simulink model "Imduction_Motor_Model_main"  (R2024a)
settings: Solver=VariableStepAuto  StartTime=0.0  StopTime=15  RelTol=1e-3
libraries: POWER_FACTOR x2, spsPower3phInstantaneousLib x2, spsThreePhaseVIMeasurementLib x2, spsAsynchronousMachineSIUnitsLib x1, Auto_transformer_Starter x1, spsGroundLib x1, Over_Voltage_Protection_Relay x1, Over_Current_Protection_Relay x1, Random_Torque_signal_Generator x1, spsThreePhaseProgrammableVoltageSourceLib x1, spspowerguiLib x1
settings Model: Creator=gshma  LastModifiedBy=gshma

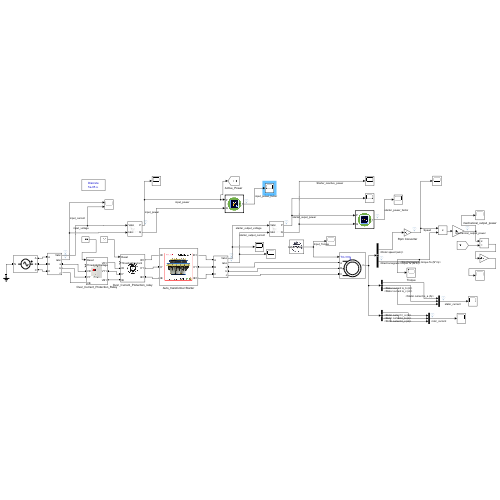
[thumbnail: Simulink's stored preview of the top-level diagram]
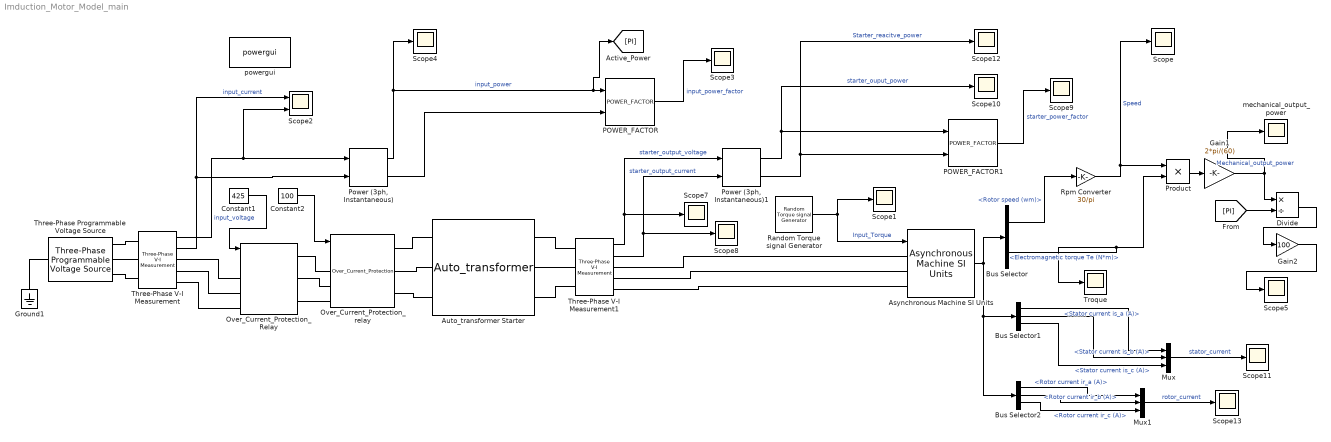
== system Imduction_Motor_Model_main ==
  Asynchronous Machine SI Units : spsAsynchronousMachineSIUnitsLib/Asynchronous Machine SI Units  RotorType=Squirrel-cage  PresetModel="15:  5.4 HP (4KW)   400 V  50Hz 1430 RPM"  MechanicalLoad=Torque Tm  ShowDetailedParameters=on  ReferenceFrame=Rotor  Units=SI  MeasurementBus=off  NominalParameters=[4000 400 50]  VoltageRatio=1  Stator=[1.405 0.005839]  Rotor=[1.395 0.005839]  Cage1=[0.4155 0.002066]  Cage2=[0.4168 0.0003495]  Lm=0.1722  Mechanical=[0.0131 0.002985 2]  PolePairs=2  InitialConditions=[0.05 0 0 0 0 0 0 0]  SimulateSaturation=off  Saturation=[14.03593122, 27.81365428, 53.79336849, 72.68890987, 97.98006896, 148.6815601, 215.7428561, 302.9841135, 428.7778367 ; 230, 322, 414, 460, 506, 552, 598, 644, 690]  LoadFlowParameters=1492000  TsPowergui=0  TsBlock=-1  IterativeModel=Trapezoidal non iterative  IterativeDiscreteModel=Trapezoidal non iterative  Pmec=1.492e+006
  Auto_transformer Starter : Auto_transformer_Starter/Auto_transformer  SystemSampleTime=-1  VariantActivationTime=update diagram  AllowFlexibleInterface=on  Latency=0  AutoFrameSizeCalculation=off
  Bus Selector : BusSelector  OutputSignals=Mechanical.Rotor speed (wm),Mechanical.Electromagnetic torque Te (N*m)
  Bus Selector1 : BusSelector  OutputSignals=Stator measurements.Stator current is_a (A),Stator measurements.Stator current is_b (A),Stator measurements.Stator current is_c (A)
  Bus Selector2 : BusSelector  OutputSignals=Rotor measurements.Rotor current ir_a (A),Rotor measurements.Rotor current ir_b (A),Rotor measurements.Rotor current ir_c (A)
  Constant1 : Constant  Value=425  SampleTime=0.001
  Constant2 : Constant  Value=100  SampleTime=0.001
  Divide : Product  Inputs=*/  RndMeth=Zero  SaturateOnIntegerOverflow=on
  Gain1 : Gain  Gain=2*pi/(60)
  Gain2 : Gain  Gain=100
  Ground1 : spsGroundLib/Ground  LConnTagsString=a
  Mux : Mux  Inputs=3
  Mux1 : Mux  Inputs=3
  Over_Current_Protection_Relay : Over_Voltage_Protection_Relay/Over_Current_Protection  SystemSampleTime=-1  VariantActivationTime=update diagram  AllowFlexibleInterface=on  Latency=0  AutoFrameSizeCalculation=off
  Over_Current_Protection_relay : Over_Current_Protection_Relay/Over_Current_Protection  SystemSampleTime=-1  VariantActivationTime=update diagram  AllowFlexibleInterface=on  Latency=0  AutoFrameSizeCalculation=off
  POWER_FACTOR : POWER_FACTOR/POWER_FACTOR  SystemSampleTime=-1  VariantActivationTime=update diagram  AllowFlexibleInterface=on  Latency=0  AutoFrameSizeCalculation=off
  POWER_FACTOR1 : POWER_FACTOR/POWER_FACTOR  SystemSampleTime=-1  VariantActivationTime=update diagram  AllowFlexibleInterface=on  Latency=0  AutoFrameSizeCalculation=off
  "Power (3ph, Instantaneous)" : spsPower3phInstantaneousLib/Power (3ph, Instantaneous)
  "Power (3ph, Instantaneous)1" : spsPower3phInstantaneousLib/Power (3ph, Instantaneous)
  Product : Product
  Random Torque signal Generator : Random_Torque_signal_Generator/Random Torque signal Generator  SystemSampleTime=-1  VariantActivationTime=update diagram  AllowFlexibleInterface=on  Latency=0  AutoFrameSizeCalculation=off
  Rpm Converter : Gain  Gain=30/pi
  Scope{,1,3..5,7..13} (12 alike) : Scope
  Scope2 : Scope  NumInputPorts=2
  Three-Phase Programmable Voltage Source : spsThreePhaseProgrammableVoltageSourceLib/Three-Phase Programmable Voltage Source  PositiveSequence="[400  0 50]"  VariationEntity=None  VariationType=Table of time-amplitude pairs  VariationTypeAlt=Step  VariationStep=0.5  VariationRate=10  VariationMagnitude=0.3  VariationFrequency=2  VariationTiming=[1 2]  VariationPhaseA=off  Amplitudes=[1 0.8 1.2 1.0]  TimeValues=[0 0.1 0.15 0.2]  HarmonicGeneration=off  HarmonicA=[3 0.2 -25 0]  HarmonicB=[2 0.15 35 2]  Timing="[0.05  3]"  BusType=swing  Pref=0  Qref=0  Qmin=-inf  Qmax=inf
  Three-Phase V-I Measurement : spsThreePhaseVIMeasurementLib/Three-Phase V-I Measurement  VoltageMeasurement=phase-to-ground  SetLabelV=off  LabelV=Vabc  Vpu=off  VpuLL=off  CurrentMeasurement=yes  SetLabelI=off  LabelI=Iabc  Ipu=off  Pbase=100e6  Vbase=500e3  OutputType=Complex  PhasorSimulation=off  PSBequivalent=0
  Three-Phase V-I Measurement1 : spsThreePhaseVIMeasurementLib/Three-Phase V-I Measurement  VoltageMeasurement=phase-to-ground  SetLabelV=off  LabelV=Vabc  Vpu=off  VpuLL=off  CurrentMeasurement=yes  SetLabelI=off  LabelI=Iabc  Ipu=off  Pbase=100e6  Vbase=500e3  OutputType=Complex  PhasorSimulation=off  PSBequivalent=0
  Troque : Scope
  mechanical_output_power : Scope
  powergui : spspowerguiLib/powergui  Priority=1  SimulationMode=Discrete  SampleTime=50e-6  frequency=60  Iterations=50  frequencyindice=50  Pbase=100e6  ErrMax=1e-4  UnitsV=kV  UnitsW=MW  buscounter=0  FunctionMessages=off  echomessages=off  EnableUseOfTLC=off  CurrentSourceSwitches=off  DisableSnubberDevices=off  DisableRonSwitches=off  DisableVfSwitches=off  DisplayEquations=off  AutomaticDiscreteSolvers=off  SolverType=Tustin/Backward Euler (TBE)  Interpol=off  ExternalGateDelay=off  methode=off  Ts=100  x0status=blocks  SPID=on  SwTol=0  HookPort=off  NonlinearTolerance=1e-4  nMaxIteration=100  ContinueOnMaxIteration=off  RestoreLinks=warning  ResistiveCurrentMeasurement=off  Frange=[0:2:500]  Ylog=off  Xlog=on  ShowGrid=off  save=off  variable=ZData  structure=0  ZoomFFT=off  StartTime=0.0  cycles=1  DisplayStyle=1  fundamental=60  FreqAxis=off  MaxFrequency=1000  frequencyindicesteady=1  RmsSteady=1  display=off
  wires:
  Random Torque signal Generator/1 -> Asynchronous Machine SI Units/1, Scope1/1  "Input_Torque"
  Three-Phase V-I Measurement/1 -> "Power (3ph, Instantaneous)"/1, Scope2/2  "input_voltage"
  Three-Phase V-I Measurement/2 -> "Power (3ph, Instantaneous)"/2, Scope2/1  "input_current"
  Asynchronous Machine SI Units/1 -> Bus Selector/1, Bus Selector2/1, Bus Selector1/1
  Bus Selector/1 -> Rpm Converter/1  "<Rotor speed (wm)>"
  Rpm Converter/1 -> Scope/1, Product/1  "Speed"
  Bus Selector/2 -> Troque/1, Product/2  "<Electromagnetic torque Te (N*m)>"
  "Power (3ph, Instantaneous)"/1 -> POWER_FACTOR/1, [PI], Scope4/1  "input_power"
  "Power (3ph, Instantaneous)"/2 -> POWER_FACTOR/2
  POWER_FACTOR/1 -> Scope3/1  "input_power_factor"
  Product/1 -> Gain1/1
  Gain1/1 -> Divide/1, mechanical_output_power/1  "Mechanical_output_power"
  [PI] -> Divide/2
  Divide/1 -> Gain2/1
  Gain2/1 -> Scope5/1
  Three-Phase V-I Measurement1/2 -> Scope8/1, "Power (3ph, Instantaneous)1"/2  "starter_output_current"
  POWER_FACTOR1/1 -> Scope9/1  "starter_power_factor"
  "Power (3ph, Instantaneous)1"/1 -> Scope10/1, POWER_FACTOR1/1  "starter_ouput_power"
  Three-Phase V-I Measurement1/1 -> Scope7/1, "Power (3ph, Instantaneous)1"/1  "starter_output_voltage"
  "Power (3ph, Instantaneous)1"/2 -> Scope12/1, POWER_FACTOR1/2  "Starter_reacitve_power"
  Constant1/1 -> Over_Current_Protection_Relay/1
  Constant2/1 -> Over_Current_Protection_relay/1
  Bus Selector1/1 -> Mux/1  "<Stator current is_a (A)>"
  Bus Selector1/2 -> Mux/2  "<Stator current is_b (A)>"
  Bus Selector1/3 -> Mux/3  "<Stator current is_c (A)>"
  Mux/1 -> Scope11/1  "stator_current"
  Bus Selector2/3 -> Mux1/3  "<Rotor current ir_c (A)>"
  Bus Selector2/1 -> Mux1/1  "<Rotor current ir_a (A)>"
  Bus Selector2/2 -> Mux1/2  "<Rotor current ir_b (A)>"
  Mux1/1 -> Scope13/1  "rotor_current"
  connections:
  Ground1/LConn1 -- Three-Phase Programmable Voltage Source/LConn1
  Three-Phase Programmable Voltage Source/RConn1 -- Three-Phase V-I Measurement/LConn1
  Three-Phase Programmable Voltage Source/RConn2 -- Three-Phase V-I Measurement/LConn2
  Three-Phase Programmable Voltage Source/RConn3 -- Three-Phase V-I Measurement/LConn3
  Three-Phase V-I Measurement1/RConn1 -- Asynchronous Machine SI Units/LConn1
  Three-Phase V-I Measurement1/RConn2 -- Asynchronous Machine SI Units/LConn2
  Three-Phase V-I Measurement1/RConn3 -- Asynchronous Machine SI Units/LConn3
  Over_Current_Protection_Relay/LConn1 -- Three-Phase V-I Measurement/RConn1
  Over_Current_Protection_Relay/LConn2 -- Three-Phase V-I Measurement/RConn2
  Over_Current_Protection_Relay/LConn3 -- Three-Phase V-I Measurement/RConn3
  Over_Current_Protection_relay/LConn1 -- Over_Current_Protection_Relay/RConn1
  Over_Current_Protection_Relay/RConn2 -- Over_Current_Protection_relay/LConn2
  Over_Current_Protection_Relay/RConn3 -- Over_Current_Protection_relay/LConn3
  Auto_transformer Starter/LConn1 -- Over_Current_Protection_relay/RConn1
  Auto_transformer Starter/LConn2 -- Over_Current_Protection_relay/RConn2
  Auto_transformer Starter/LConn3 -- Over_Current_Protection_relay/RConn3
  Auto_transformer Starter/RConn1 -- Three-Phase V-I Measurement1/LConn1
  Auto_transformer Starter/RConn2 -- Three-Phase V-I Measurement1/LConn2
  Auto_transformer Starter/RConn3 -- Three-Phase V-I Measurement1/LConn3
